simulink model "Logic2method"  (R2017a)
settings: Solver=FixedStepDiscrete  StartTime=0.0  StopTime=0.02  FixedStep=2e-6  MaxStep=1e-4  RelTol=1e-3
undefined symbols (not defined in the file): DiscIntNeverNeededParam
libraries: powerlib_meascontrol x1, powerlib x1
settings Model: Creator=mayartmal  LastModifiedBy=mayartmal

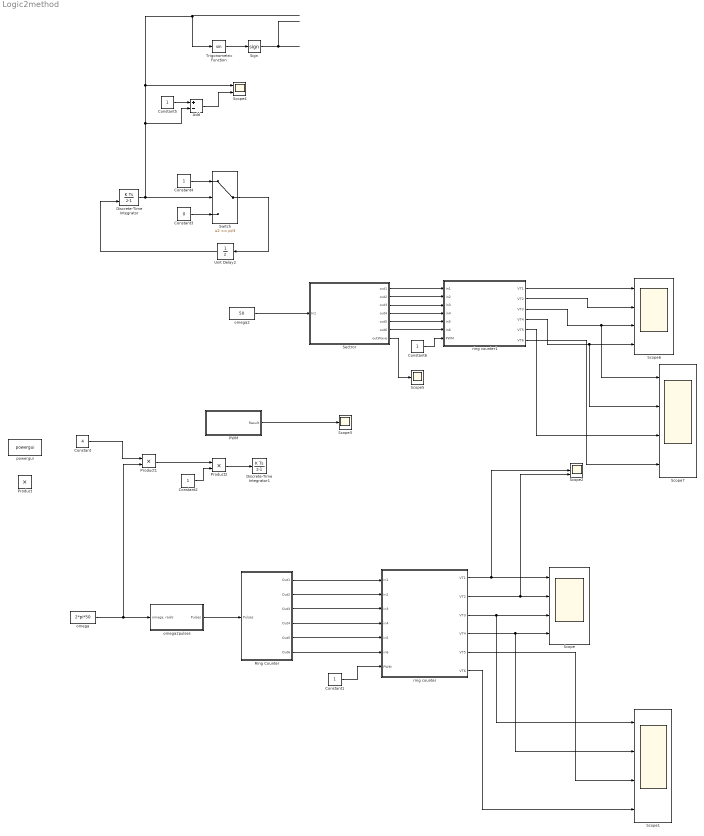
== system Logic2method ==
  Add : Sum  Inputs=+-
  Constant : Constant  Value=4
  Constant{1..2,4..6} (5 alike) : Constant
  Constant3 : Constant  Value=0
  Discrete-Time Integrator : DiscreteIntegrator  gainval=1  ExternalReset=rising  InitialConditionSetting=State (most efficient)  SampleTime=-1  ICPrevOutput=DiscIntNeverNeededParam  ICPrevScaledInput=DiscIntNeverNeededParam
  Discrete-Time Integrator1 : DiscreteIntegrator  gainval=1  InitialConditionSetting=State (most efficient)  SampleTime=-1  ICPrevOutput=DiscIntNeverNeededParam  ICPrevScaledInput=DiscIntNeverNeededParam
  PWM : Subsystem
  Product : Product
  Product1 : Product
  Product2 : Product
  Ring Counter : Subsystem
  Scope{,1,6..7} (4 alike) : Scope  NumInputPorts=4
  Scope2 : Scope  NumInputPorts=3
  Scope3 : Scope
  Scope4 : Scope  NumInputPorts=2
  Scope5 : Scope
  Sectror : Subsystem
  Sign : Signum
  Switch : Switch  Threshold=pi/3
  Trigonometric Function : Trigonometry
  Unit Delay2 : UnitDelay  SampleTime=-1
  omega : Constant  Value=2*pi*50
  omega2 : Constant  Value=50
  omega2pulses : Subsystem
  powergui : powerlib/powergui  Priority=1  SimulationMode=Discrete  SampleTime=2e-6  frequency=60  Iterations=50  frequencyindice=0  Pbase=100e6  ErrMax=1e-4  UnitsV=kV  UnitsW=MW  buscounter=0  FunctionMessages=off  echomessages=off  EnableUseOfTLC=off  CurrentSourceSwitches=off  DisableSnubberDevices=off  DisableRonSwitches=off  DisableVfSwitches=off  DisplayEquations=off  SolverType=Tustin/Backward Euler (TBE)  Interpol=off  ExternalGateDelay=off  methode=off  Ts=100  x0status=blocks  SPID=off  SwTol=0  HookPort=off  RestoreLinks=warning  ResistiveCurrentMeasurement=off  Frange=[0:2:500]  Ylog=off  Xlog=on  ShowGrid=off  save=off  variable=ZData  structure=0  ZoomFFT=off  StartTime=0.0  cycles=1  DisplayStyle=1  fundamental=60  FreqAxis=off  MaxFrequency=1000  frequencyindicesteady=1  RmsSteady=1  display=off
  ring counter : MATLAB Function  TreatAsAtomicUnit=on
  ring counter1 : MATLAB Function  TreatAsAtomicUnit=on
  wires:
  omega2pulses/1(Pulses) -> Ring Counter/1(Pulses)
  Constant1/1 -> ring counter/7(PWM)
  ring counter/1(VT1) -> Scope2/2, Scope/1
  Ring Counter/3(Out3) -> ring counter/3(in3)
  Ring Counter/4(Out4) -> ring counter/4(in4)
  Ring Counter/2(Out2) -> ring counter/2(in2)
  Ring Counter/5(Out5) -> ring counter/5(in5)
  Ring Counter/1(Out1) -> ring counter/1(in1)
  Ring Counter/6(Out6) -> ring counter/6(in6)
  ring counter/2(VT2) -> Scope2/3, Scope/2
  ring counter/3(VT3) -> Scope1/1, Scope/3
  ring counter/4(VT4) -> Scope1/2, Scope/4
  ring counter/5(VT5) -> Scope1/3
  ring counter/6(VT6) -> Scope1/4
  omega/1 -> Product1/2, omega2pulses/1("omega, rad/s")
  Constant/1 -> Product1/1
  Discrete-Time Integrator/1 -> Switch/2, Trigonometric Function/1, Scope4/1, Add/2
  Constant5/1 -> Add/1
  Add/1 -> Scope4/2
  Constant3/1 -> Switch/3
  Switch/1 -> Unit Delay2/1
  Constant4/1 -> Switch/1
  Sign/1 -> ?
  Trigonometric Function/1 -> Sign/1
  Unit Delay2/1 -> Discrete-Time Integrator/2
  Product2/1 -> Discrete-Time Integrator1/1
  Product1/1 -> Product2/1
  Constant2/1 -> Product2/2
  PWM/1(Result) -> Scope3/1
  omega2/1 -> Sectror/1(In1)
  Sectror/5(out5) -> ring counter1/5(in5)
  Sectror/4(out4) -> ring counter1/4(in4)
  Sectror/6(out6) -> ring counter1/6(in6)
  Sectror/3(out3) -> ring counter1/3(in3)
  Sectror/2(out2) -> ring counter1/2(in2)
  Sectror/1(out1) -> ring counter1/1(in1)
  Sectror/7(outWave) -> Scope5/1
  Constant6/1 -> ring counter1/7(PWM)
  ring counter1/1(VT1) -> Scope6/1
  ring counter1/2(VT2) -> Scope6/2
  ring counter1/4(VT4) -> Scope7/2, Scope6/4
  ring counter1/3(VT3) -> Scope7/1, Scope6/3
  ring counter1/5(VT5) -> Scope7/3
  ring counter1/6(VT6) -> Scope7/4

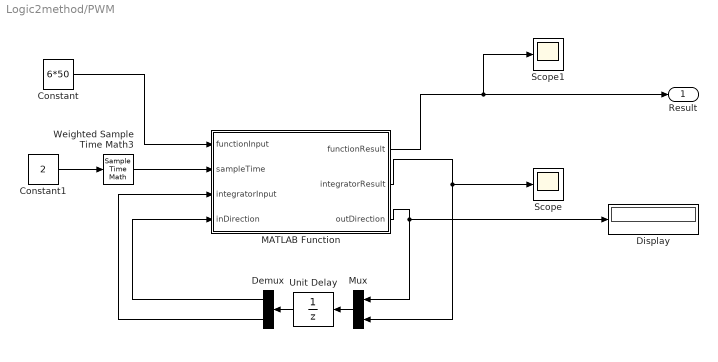
== system Logic2method/PWM ==
  Constant : Constant  Value=6*50
  Constant1 : Constant  Value=2
  Demux : Demux  Outputs=2
  Display : Display
  MATLAB Function : MATLAB Function  TreatAsAtomicUnit=on
  Mux : Mux  Inputs=2
  Scope : Scope
  Scope1 : Scope
  Unit Delay : UnitDelay  SampleTime=-1
  Weighted Sample Time Math3 : SampleTimeMath  TsampMathOp=*
  Result : Outport
  wires:
  Demux/2 -> MATLAB Function/3(integratorInput)
  MATLAB Function/2(integratorResult) -> Mux/2, Scope/1
  MATLAB Function/1(functionResult) -> Scope1/1, Result/1
  Weighted Sample Time Math3/1 -> MATLAB Function/2(sampleTime)
  Constant/1 -> MATLAB Function/1(functionInput)
  Demux/1 -> MATLAB Function/4(inDirection)
  MATLAB Function/3(outDirection) -> Mux/1, Display/1
  Constant1/1 -> Weighted Sample Time Math3/1
  Unit Delay/1 -> Demux/1
  Mux/1 -> Unit Delay/1

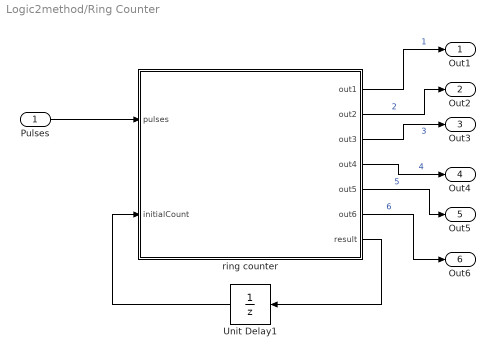
== system Logic2method/Ring Counter ==
  Pulses : Inport
  Unit Delay1 : UnitDelay  InitialCondition=1  SampleTime=-1
  ring counter : MATLAB Function  TreatAsAtomicUnit=on
  Out1 : Outport
  Out2 : Outport  Port=2
  Out3 : Outport  Port=3
  Out4 : Outport  Port=4
  Out5 : Outport  Port=5
  Out6 : Outport  Port=6
  wires:
  Unit Delay1/1 -> ring counter/2(initialCount)
  ring counter/7(result) -> Unit Delay1/1
  ring counter/3(out3) -> Out3/1  "3"
  ring counter/5(out5) -> Out5/1  "5"
  ring counter/4(out4) -> Out4/1  "4"
  ring counter/2(out2) -> Out2/1  "2"
  ring counter/6(out6) -> Out6/1  "6"
  Pulses/1 -> ring counter/1(pulses)
  ring counter/1(out1) -> Out1/1  "1"

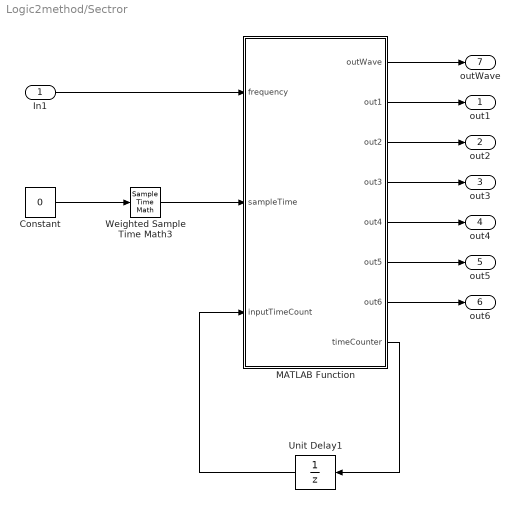
== system Logic2method/Sectror ==
  In1 : Inport
  Constant : Constant  Value=0
  MATLAB Function : MATLAB Function  TreatAsAtomicUnit=on
  Unit Delay1 : UnitDelay  SampleTime=-1
  Weighted Sample Time Math3 : SampleTimeMath  TsampMathOp=Ts Only
  out1 : Outport
  out2 : Outport  Port=2
  out3 : Outport  Port=3
  out4 : Outport  Port=4
  out5 : Outport  Port=5
  out6 : Outport  Port=6
  outWave : Outport  Port=7
  wires:
  Weighted Sample Time Math3/1 -> MATLAB Function/2(sampleTime)
  Unit Delay1/1 -> MATLAB Function/3(inputTimeCount)
  MATLAB Function/8(timeCounter) -> Unit Delay1/1
  In1/1 -> MATLAB Function/1(frequency)
  MATLAB Function/3(out2) -> out2/1
  MATLAB Function/7(out6) -> out6/1
  MATLAB Function/1(outWave) -> outWave/1
  MATLAB Function/4(out3) -> out3/1
  MATLAB Function/5(out4) -> out4/1
  MATLAB Function/2(out1) -> out1/1
  MATLAB Function/6(out5) -> out5/1
  Constant/1 -> Weighted Sample Time Math3/1

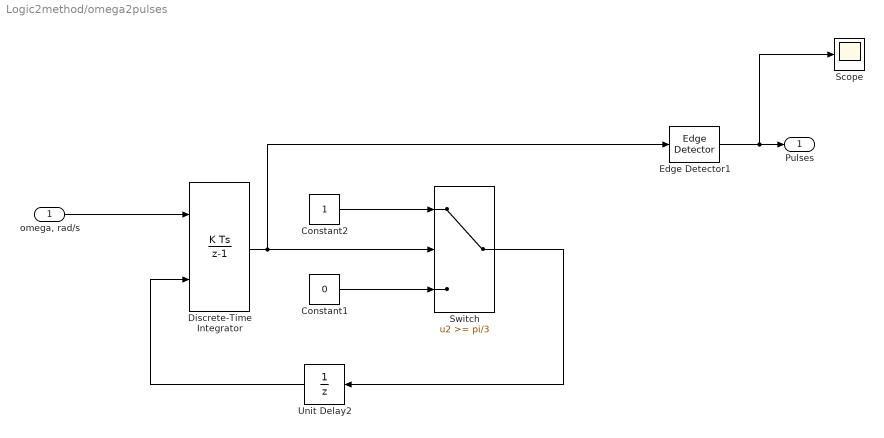
== system Logic2method/omega2pulses ==
  "omega, rad/s" : Inport
  Constant1 : Constant  Value=0
  Constant2 : Constant
  Discrete-Time Integrator : DiscreteIntegrator  ExternalReset=rising  InitialConditionSetting=State (most efficient)  SampleTime=-1  ICPrevOutput=DiscIntNeverNeededParam  ICPrevScaledInput=DiscIntNeverNeededParam
  Edge Detector1 : powerlib_meascontrol/Logic/Edge Detector  model=Falling  ic=0  Ts=-1
      settings: SourceProductName=Simscape Power Systems  SourceProductBaseCode=PS
  Scope : Scope
  Switch : Switch  Threshold=pi/3
  Unit Delay2 : UnitDelay  SampleTime=-1
  Pulses : Outport
  wires:
  Switch/1 -> Unit Delay2/1
  Discrete-Time Integrator/1 -> Edge Detector1/1, Switch/2
  Unit Delay2/1 -> Discrete-Time Integrator/2
  Constant1/1 -> Switch/3
  Constant2/1 -> Switch/1
  Edge Detector1/1 -> Scope/1, Pulses/1
  "omega, rad/s"/1 -> Discrete-Time Integrator/1

== matlab function Logic2method/ring counter ==
  data: in1 input; in2 input; in3 input; in4 input; in5 input; in6 input; VT1 output; PWM input; VT2 output; VT3 output; VT4 output; VT5 output; VT6 output
function [VT1, VT2, VT3, VT4, VT5, VT6] = fcn(in1, in2, in3, in4, in5, in6, PWM)

VT1 = in1 | (in2 & PWM) | in3 |(in5 & (~PWM));
VT2 = (in2 & (~PWM)) | in4 | (in5 & PWM) | in6;

VT3 = in3 | (in4 & PWM) | in5 |(in1 & (~PWM));
VT4 = (in4 & (~PWM)) | in6 | (in1 & PWM) | in2;

VT5 = in5 | (in6 & PWM) | in1 |(in3 & (~PWM));
VT6 = (in6 & (~PWM)) | in2 | (in3 & PWM) | in4;



end

== matlab function Logic2method/PWM/MATLAB Function ==
  data: functionResult output; functionInput input; sampleTime input; integratorResult output; integratorInput input; inDirection input; outDirection output
function [functionResult, integratorResult, outDirection]= fcn(functionInput, sampleTime, integratorInput, inDirection)
if inDirection == 0
    integratorResult = integratorInput + sampleTime;
elseif inDirection == 1
    integratorResult = integratorInput - sampleTime;
else
    integratorResult = integratorInput;
end

functionResult = functionInput * integratorResult;

if functionResult >= 1
    outDirection = 1;
elseif functionResult <= 0
    outDirection = 0;
else 
    outDirection = inDirection;
end




end

== matlab function Logic2method/Sectror/MATLAB Function ==
  data: outWave output; out1 output; out2 output; out3 output; out4 output; out5 output; out6 output; frequency input; sampleTime input; timeCounter output; inputTimeCount input
function [outWave, out1, out2, out3, out4, out5, out6, timeCounter]= fcn(frequency, sampleTime, inputTimeCount)

period = 1 / frequency;
halfPeriod = period * 0.5;
oneSixthPeriod = period / 6;



if inputTimeCount <= halfPeriod
    waveSign = 0;
elseif inputTimeCount > halfPeriod
    waveSign = 1;
else
    waveSign = 0;
end

timeCounter = inputTimeCount + sampleTime;
if timeCounter >= period
    timeCounter = 0;
end





if waveSign == 0
    outWave = 1;
elseif waveSign == 1
    outWave = -1;
else
    outWave = 0;
end


%out1
if (inputTimeCount >= 0) && (inputTimeCount < oneSixthPeriod)
       out1 = 1;
else
       out1 = 0;
end

%out2
if (inputTimeCount >= oneSixthPeriod) && (inputTimeCount < 2 * oneSixthPeriod)
       out2 = 1;
else
       out2 = 0;
end

%out3
if (inputTimeCount >= 2 * oneSixthPeriod) && (inputTimeCount < 3 * oneSixthPeriod)
       out3 = 1;
else
       out3 = 0;
end


%out4
if (inputTimeCount >= 3 * oneSixthPeriod) && (inputTimeCount < 4 * oneSixthPeriod)
       out4 = 1;
else
       out4 = 0;
end

%out5
if (inputTimeCount >= 4 * oneSixthPeriod) && (inputTimeCount < 5 * oneSixthPeriod)
       out5 = 1;
else
       out5 = 0;
end

%out6
if (inputTimeCount >= 5 * oneSixthPeriod) && (inputTimeCount < 6 * oneSixthPeriod)
       out6 = 1;
else
       out6 = 0;
end



end

== matlab function Logic2method/Ring Counter/ring counter ==
  data: pulses input; out1 output; out2 output; initialCount input; out3 output; out4 output; out5 output; out6 output; result output
function [out1, out2, out3, out4, out5, out6, result] = fcn(pulses, initialCount)
if pulses == 1 
   result = initialCount + 1;
   if result >= 7
       result = 1;
   end        
else   
   result = initialCount;
end

%out1
if result == 1
       out1 = 1;
else
       out1 = 0;
end
%%out2
if result == 2
       out2 = 1;
else
       out2 = 0;
end
%out3
if result == 3
       out3 = 1;
else
       out3 = 0;
end
%out4
if result == 4
       out4 = 1;
else
       out4 = 0;
end
%out5
if result == 5
       out5 = 1;
else
       out5 = 0;
end 
%out6
if result == 6
       out6 = 1;
else
       out6 = 0;
end


end

== matlab function Logic2method/ring counter1 ==
  data: in1 input; in2 input; in3 input; in4 input; in5 input; in6 input; VT1 output; PWM input; VT2 output; VT3 output; VT4 output; VT5 output; VT6 output
function [VT1, VT2, VT3, VT4, VT5, VT6] = fcn(in1, in2, in3, in4, in5, in6, PWM)

VT1 = in1 | (in2 & PWM) | in3 |(in5 & (~PWM));
VT2 = (in2 & (~PWM)) | in4 | (in5 & PWM) | in6;

VT3 = in3 | (in4 & PWM) | in5 |(in1 & (~PWM));
VT4 = (in4 & (~PWM)) | in6 | (in1 & PWM) | in2;

VT5 = in5 | (in6 & PWM) | in1 |(in3 & (~PWM));
VT6 = (in6 & (~PWM)) | in2 | (in3 & PWM) | in4;



end
